simulink subsystem "MPC18_nlpsol"  (R2022b)
settings: Solver=VariableStepAuto  StartTime=0.0  StopTime=10.0  RelTol=1e-3
undefined symbols (not defined in the file): param_global, param_MPC01, param_robot, param_weight_init
settings Model: Creator=emu  LastModifiedBy=emu
settings OptimizationCC: ReuseModelBlockBuffer=on

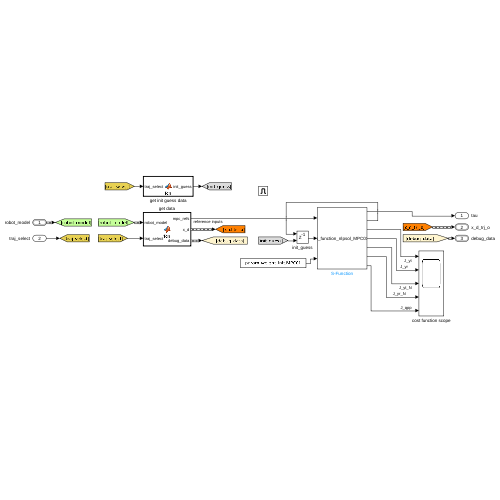
[thumbnail: Simulink's stored preview of the top-level diagram]
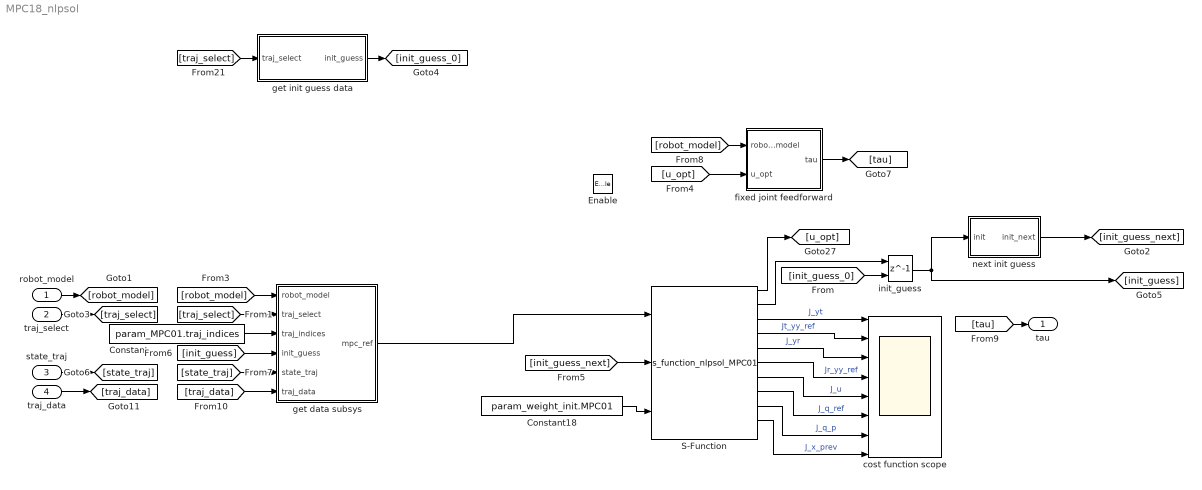
== system MPC18_nlpsol ==
  robot_model : Inport  OutDataTypeStr=Bus: robot_model
  traj_select : Inport  Port=2
  state_traj : Inport  Port=3  OutDataTypeStr=Bus: state_traj_bus
  traj_data : Inport  Port=4  OutDataTypeStr=Bus: traj_data_bus
  Enable : EnablePort
  Constant : Constant  Value=param_MPC01.traj_indices
  Constant18 : Constant  Value=param_weight_init.MPC01  VectorParams1D=off
  S-Function : S-Function  FunctionName=s_function_nlpsol_MPC01  Parameters='s_functions/fr3_no_hand_6dof/MPC01.casadi', 'MPC01'  SFunctionModules='MPC01'  SFunctionDeploymentMode=off  EnableBusSupport=off
  cost function scope : Scope  NumInputPorts=8
  fixed joint feedforward : MATLAB Function  TreatAsAtomicUnit=on
  get data subsys : Subsystem
  get init guess data : MATLAB Function  TreatAsAtomicUnit=on
  init_guess : Delay  DelayLength=1  InitialConditionSource=Input port  InitialCondition=1
      settings: InputPortMap=u0,p4
  next init guess : MATLAB Function  TreatAsAtomicUnit=on
  tau : Outport
  wires:
  [init_guess_next] -> S-Function/2
  S-Function/1 -> [u_opt]
  next init guess/1(init_next) -> [init_guess_next]
  init_guess/1 -> [init_guess], next init guess/1(init)
  [tau] -> tau/1
  fixed joint feedforward/1(tau) -> [tau]
  [robot_model] -> fixed joint feedforward/1(robot_model)
  [u_opt] -> fixed joint feedforward/2(u_opt)
  S-Function/2 -> init_guess/1
  [init_guess_0] -> init_guess/2
  traj_select/1 -> [traj_select]
  get init guess data/1(init_guess) -> [init_guess_0]
  [traj_select] -> get init guess data/1(traj_select)
  Constant18/1 -> S-Function/3
  robot_model/1 -> [robot_model]
  [robot_model] -> get data subsys/1(robot_model)
  [traj_select] -> get data subsys/2(traj_select)
  Constant/1 -> get data subsys/3(traj_indices)
  [init_guess] -> get data subsys/4(init_guess)
  get data subsys/1(mpc_ref) -> S-Function/1
  state_traj/1 -> [state_traj]
  [state_traj] -> get data subsys/5(state_traj)
  traj_data/1 -> [traj_data]
  [traj_data] -> get data subsys/6(traj_data)
  S-Function/8 -> cost function scope/6  "J_q_ref"
  S-Function/9 -> cost function scope/7  "J_q_p"
  S-Function/5 -> cost function scope/3  "J_yr"
  S-Function/4 -> cost function scope/2  "Jt_yy_ref"
  S-Function/6 -> cost function scope/4  "Jr_yy_ref"
  S-Function/3 -> cost function scope/1  "J_yt"
  S-Function/10 -> cost function scope/8  "J_x_prev"
  S-Function/7 -> cost function scope/5  "J_u"

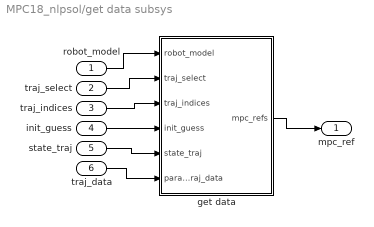
== system MPC18_nlpsol/get data subsys ==
  robot_model : Inport  OutDataTypeStr=Bus: robot_model
  traj_select : Inport  Port=2
  traj_indices : Inport  Port=3
  init_guess : Inport  Port=4
  state_traj : Inport  Port=5  OutDataTypeStr=Bus: state_traj_bus
  traj_data : Inport  Port=6  OutDataTypeStr=Bus: traj_data_bus
  get data : MATLAB Function  TreatAsAtomicUnit=on
  mpc_ref : Outport
  wires:
  traj_data/1 -> get data/6(param_traj_data)
  state_traj/1 -> get data/5(state_traj)
  init_guess/1 -> get data/4(init_guess)
  robot_model/1 -> get data/1(robot_model)
  traj_select/1 -> get data/2(traj_select)
  traj_indices/1 -> get data/3(traj_indices)
  get data/1(mpc_refs) -> mpc_ref/1

== matlab function MPC18_nlpsol/fixed joint feedforward ==
  data: robot_model input Bus: robot_model; tau output; u_opt input; param_robot parameter
function tau= fcn(robot_model, u_opt, param_robot)

n = param_robot.n_DOF;

if size(u_opt, 2) ~= 0 && size(u_opt, 1) ~= 1
    n_indices = param_robot.n_indices;
    n_red = param_robot.n_red;

    tau_red = u_opt(1:n_red);

    M = robot_model.M;      % inertia matrix
    g = robot_model.g;

    C_rnea = robot_model.C_rnea; % C_rnea(q, q_p) = C(q, q_p)q_p + g(q) = n(q, q_p)

    Cqp = C_rnea - g;
    M_red = M(n_indices, n_indices);

    q_pp_red = M_red\(tau_red - Cqp(n_indices)); % gravity is ignored here
    q_pp = zeros(n, 1);
    q_pp(n_indices) = q_pp_red;

    tau = M*q_pp + Cqp;
else
    tau = zeros(n,1);
end

== matlab function MPC18_nlpsol/get data subsys/get data ==
  settings: updateMethod=DISCRETE  sampleTime=param_global.Ta
  data: mpc_refs output; robot_model input Bus: robot_model; traj_select input; traj_indices input; init_guess input; state_traj input Bus: state_traj_bus; param_robot parameter; param_traj_data input
function mpc_refs  = fcn(robot_model, traj_select, traj_indices, init_guess, state_traj, param_robot, param_traj_data)
persistent cnt;
persistent run_flag;

if(isempty(cnt))
    cnt = 1;
    run_flag = 0;
end

n_indices = param_robot.n_indices;
traj_indices = traj_indices + (cnt-1);
N_MPC = length(traj_indices)-1;
n_red = param_robot.n_red;

% Parameters
q    = robot_model.q;      % generalized coordinates
q_p  = robot_model.q_p;  % time derivative of generalized coordinates

x_k = [q(n_indices);q_p(n_indices)];

% Assemble vector of recieved output measurements
p_d     = param_traj_data.p_d(   1:3, traj_indices, traj_select);
q_d     = param_traj_data.q_d(   1:4, traj_indices, traj_select);

y_d = [p_d; q_d];

%% Reference out
N_u = n_red*N_MPC;
N_x = 2*n_red * (N_MPC+1);

if(cnt == 1)
    u_prev = zeros(N_u,1);
else
    u_prev = init_guess(1:N_u);
end
x_k_prev = init_guess(1+N_u : N_u+N_x);
mpc_refs = [x_k(:); y_d(:); x_k_prev(:); u_prev(:)];

[run_flag, cnt] = update_traj_cnt(state_traj, run_flag, cnt, param_traj_data.N);

== matlab function MPC18_nlpsol/get init guess data ==
  data: traj_select input; param_MPC01_init_guess parameter; init_guess output
function init_guess  = fcn(traj_select, param_MPC01_init_guess)

init_guess = param_MPC01_init_guess.init_guess(traj_select,:);

== matlab function MPC18_nlpsol/next init guess ==
  data: init input; init_next output; param_MPC01 parameter; param_robot parameter; param_global parameter
function init_next = fcn(init, param_MPC01, param_robot, param_global)
param_MPC = param_MPC01;

Ta = param_global.Ta;
dt_arr = param_MPC.int_times;
N_MPC = param_MPC.N;
n_red = param_robot.n_red;
N_u = n_red * N_MPC;
N_x = (2*n_red)*(N_MPC+1);

N = 0;

u_idx = N + [1:N_u];       N = N + length(u_idx);
u_idx_2d = reshape(u_idx, n_red, N_MPC);
u_idx_2d(:, 1:end-1) = u_idx_2d(:, 2:end);

x_idx = N + [1:N_x];       N = N + length(x_idx);
x_idx_2d = reshape(x_idx, 2*n_red, (N_MPC+1));
x_idx_2d(:, 1:end-1) = x_idx_2d(:, 2:end);

%q_idx = N + [1:n_red];     N = N + length(q_idx);
%
%lam_u_idx = N + [1:N_u];   N = N + length(lam_u_idx);
%lam_u_idx_2d = reshape(lam_u_idx, n_red, N_MPC);
%lam_u_idx_2d(:, 1:end-1) = lam_u_idx_2d(:, 2:end);
%
%lam_x_idx = N + [1:N_x];   N = N + length(lam_x_idx);
%lam_x_idx_2d = reshape(lam_x_idx, 2*n_red, (N_MPC+1));
%lam_x_idx_2d(:, 1:end-1) = lam_x_idx_2d(:, 2:end);
%
%lam_q_idx = N + [1:n_red]; N = N + length(lam_q_idx);
%
%lam_g_x_idx = N + [1:N_x]; N = N + length(lam_g_x_idx);
%lam_g_idx_2d = reshape(lam_g_x_idx, 2*n_red, (N_MPC+1));
%lam_g_idx_2d(:, 1:end-1) = lam_g_idx_2d(:, 2:end);
%
%lam_g_q_idx = N + [1:n_red];

x_init = init(x_idx_2d);
u_init = init(u_idx_2d);

dx = (x_init(:, 2:end) - x_init(:, 1:end-1))./dt_arr;
x_next = x_init(:, 1:end-1) + dx * Ta;

du = (u_init(:, 2:end) - u_init(:, 1:end-1))./dt_arr(1:end-1);
u_next = u_init(:, 1:end-1) + du * Ta;

x_idx_m1 = x_idx_2d(:, 1:end-1);
u_idx_m1 = u_idx_2d(:, 1:end-1);

init_next = init';
%init_next = init([u_idx_2d(:); x_idx_2d(:); q_idx(:); lam_u_idx_2d(:); lam_x_idx_2d(:); lam_q_idx(:); lam_g_idx_2d(:); lam_g_q_idx(:)])';
init_next(x_idx_m1) = x_next;
init_next(u_idx_m1) = u_next;
